simulink model "Ellipse"  (R2017b)
settings: Solver=FixedStepAuto  StartTime=0.0  StopTime=10.0  RelTol=1e-3
settings Model: Creator=Eric  LastModifiedBy=dwegg
settings SolverCC: AlgebraicLoopSolver=LineSearch
settings RTWCC: SystemTargetFile=irt.tlc  TemplateMakefile=irt_default_tmf  Description=INTECRIO Real-Time Target
settings STFCustomTargetCC: TargetLangStandard=C99 (ISO)  UtilityFuncGeneration=Shared location  SystemTargetFile=irt.tlc
settings GRTTargetCC: UtilityFuncGeneration=Shared location  ParMdlRefBuildCompliant=off  CompOptLevelCompliant=off  ConcurrentExecutionCompliant=off  CombineOutputUpdateFcns=off  MatFileLogging=off  CPPClassGenCompliant=off  GRTInterface=on  UseToolchainInfoCompliant=off  GenerateASAP2=on

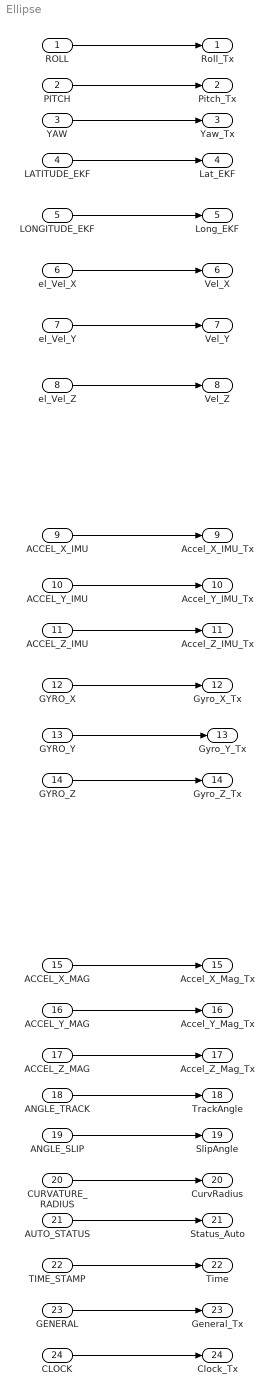
== system Ellipse ==
  ROLL : Inport
  PITCH : Inport  Port=2
  YAW : Inport  Port=3
  LATITUDE_EKF : Inport  Port=4
  LONGITUDE_EKF : Inport  Port=5
  el_Vel_X : Inport  Port=6
  el_Vel_Y : Inport  Port=7
  el_Vel_Z : Inport  Port=8
  ACCEL_X_IMU : Inport  Port=9
  ACCEL_Y_IMU : Inport  Port=10
  ACCEL_Z_IMU : Inport  Port=11
  GYRO_X : Inport  Port=12
  GYRO_Y : Inport  Port=13
  GYRO_Z : Inport  Port=14
  ACCEL_X_MAG : Inport  Port=15
  ACCEL_Y_MAG : Inport  Port=16
  ACCEL_Z_MAG : Inport  Port=17
  ANGLE_TRACK : Inport  Port=18
  ANGLE_SLIP : Inport  Port=19
  CURVATURE_RADIUS : Inport  Port=20
  AUTO_STATUS : Inport  Port=21
  TIME_STAMP : Inport  Port=22
  GENERAL : Inport  Port=23
  CLOCK : Inport  Port=24
  Roll_Tx : Outport
  Pitch_Tx : Outport  Port=2
  Yaw_Tx : Outport  Port=3
  Lat_EKF : Outport  Port=4
  Long_EKF : Outport  Port=5
  Vel_X : Outport  Port=6
  Vel_Y : Outport  Port=7
  Vel_Z : Outport  Port=8
  Accel_X_IMU_Tx : Outport  Port=9
  Accel_Y_IMU_Tx : Outport  Port=10
  Accel_Z_IMU_Tx : Outport  Port=11
  Gyro_X_Tx : Outport  Port=12
  Gyro_Y_Tx : Outport  Port=13
  Gyro_Z_Tx : Outport  Port=14
  Accel_X_Mag_Tx : Outport  Port=15
  Accel_Y_Mag_Tx : Outport  Port=16
  Accel_Z_Mag_Tx : Outport  Port=17
  TrackAngle : Outport  Port=18
  SlipAngle : Outport  Port=19
  CurvRadius : Outport  Port=20
  Status_Auto : Outport  Port=21
  Time : Outport  Port=22
  General_Tx : Outport  Port=23
  Clock_Tx : Outport  Port=24
  wires:
  CLOCK/1 -> Clock_Tx/1
  GENERAL/1 -> General_Tx/1
  TIME_STAMP/1 -> Time/1
  AUTO_STATUS/1 -> Status_Auto/1
  CURVATURE_RADIUS/1 -> CurvRadius/1
  ANGLE_SLIP/1 -> SlipAngle/1
  ANGLE_TRACK/1 -> TrackAngle/1
  ACCEL_Z_MAG/1 -> Accel_Z_Mag_Tx/1
  ACCEL_Y_MAG/1 -> Accel_Y_Mag_Tx/1
  ACCEL_X_MAG/1 -> Accel_X_Mag_Tx/1
  GYRO_Z/1 -> Gyro_Z_Tx/1
  GYRO_Y/1 -> Gyro_Y_Tx/1
  GYRO_X/1 -> Gyro_X_Tx/1
  ACCEL_Z_IMU/1 -> Accel_Z_IMU_Tx/1
  ACCEL_Y_IMU/1 -> Accel_Y_IMU_Tx/1
  ACCEL_X_IMU/1 -> Accel_X_IMU_Tx/1
  el_Vel_Z/1 -> Vel_Z/1
  el_Vel_Y/1 -> Vel_Y/1
  el_Vel_X/1 -> Vel_X/1
  LONGITUDE_EKF/1 -> Long_EKF/1
  LATITUDE_EKF/1 -> Lat_EKF/1
  YAW/1 -> Yaw_Tx/1
  PITCH/1 -> Pitch_Tx/1
  ROLL/1 -> Roll_Tx/1
